simulink model "SensorModels"  (R2018b)
settings: Solver=VariableStepAuto  StartTime=0.0  StopTime=10.0  RelTol=1e-3
libraries: simulink x5
settings Model: Creator=Andrew  LastModifiedBy=Andrew

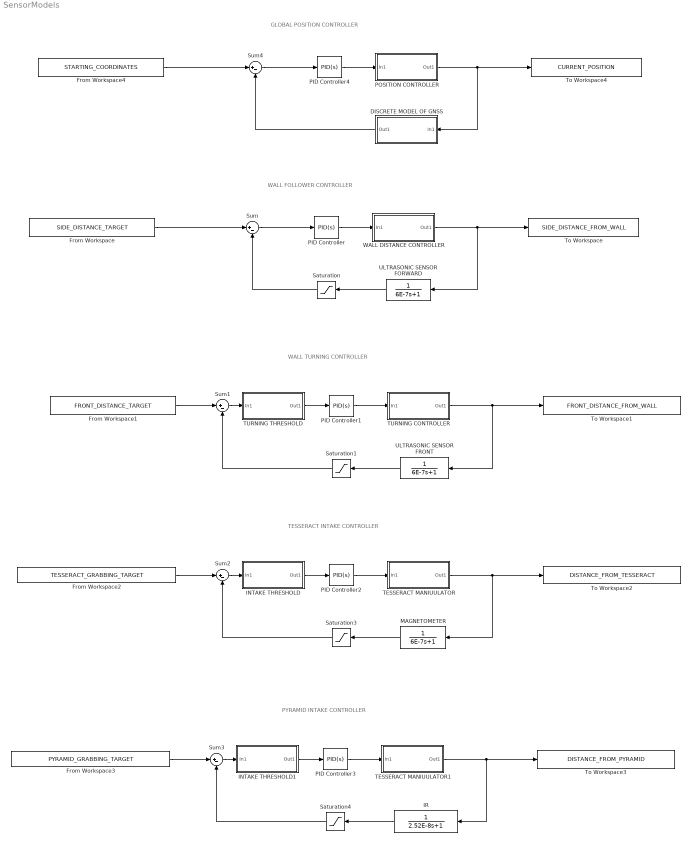
== system SensorModels ==
  note: WALL FOLLOWER CONTROLLER
  note: WALL TURNING CONTROLLER
  note: TESSERACT INTAKE CONTROLLER
  note: PYRAMID INTAKE CONTROLLER
  note: GLOBAL POSITION CONTROLLER
  DISCRETE MODEL OF GNSS : Subsystem
  From Workspace : FromWorkspace  VariableName=SIDE_DISTANCE_TARGET  SampleTime=0
  From Workspace1 : FromWorkspace  VariableName=FRONT_DISTANCE_TARGET  SampleTime=0
  From Workspace2 : FromWorkspace  VariableName=TESSERACT_GRABBING_TARGET  SampleTime=0
  From Workspace3 : FromWorkspace  VariableName=PYRAMID_GRABBING_TARGET  SampleTime=0
  From Workspace4 : FromWorkspace  VariableName=STARTING_COORDINATES  SampleTime=0
  INTAKE THRESHOLD : Subsystem
  INTAKE THRESHOLD1 : Subsystem
  IR : TransferFcn  Denominator=[2.52E-8 1]
  MAGNETOMETER : TransferFcn  Denominator=[6E-7 1]
  PID Controller{,1..4} (5 alike) : simulink/Continuous/PID Controller  Controller=PID  Form=Parallel  TimeDomain=Continuous-time  SampleTime=-1  IntegratorMethod=Forward Euler  FilterMethod=Forward Euler  ControllerParametersSource=internal  P=1  I=1  D=0  UseFilter=on  N=100  TunerSelectOption=Transfer Function Based (PID Tuner App)  InitialConditionSource=internal  InitialConditionForIntegrator=0  InitialConditionForFilter=0  DifferentiatorICPrevScaledInput=0  ExternalReset=none  TrackingMode=off  Kt=1  LimitOutput=off  UpperSaturationLimit=inf  LowerSaturationLimit=-inf  LinearizeAsGain=on  AntiWindupMode=none  Kb=1  POutMin=[]  POutMax=[]  IOutMin=[]  IOutMax=[]  DOutMin=[]  DOutMax=[]  NOutMin=[]  NOutMax=[]  SumOutMin=[]  SumOutMax=[]  SaturationOutMin=[]  SaturationOutMax=[]  PParamMin=[]  PParamMax=[]  IParamMin=[]  IParamMax=[]  DParamMin=[]  DParamMax=[]  NParamMin=[]  NParamMax=[]  KbParamMin=[]  KbParamMax=[]  KtParamMin=[]  KtParamMax=[]  KbOutMin=[]  KbOutMax=[]  KtOutMin=[]  KtOutMax=[]  IntegratorOutMin=[]  IntegratorOutMax=[]  FilterOutMin=[]  FilterOutMax=[]  SumI1OutMin=[]  SumI1OutMax=[]  SumI2OutMin=[]  SumI2OutMax=[]  SumI3OutMin=[]  SumI3OutMax=[]  SumI4OutMin=[]  SumI4OutMax=[]  SumDOutMin=[]  SumDOutMax=[]  DifferentiatorOutMin=[]  DifferentiatorOutMax=[]  FilterDiffOutCoefMin=[]  FilterDiffOutCoefMax=[]  ReciprocalOutMin=[]  ReciprocalOutMax=[]  SumDenOutMin=[]  SumDenOutMax=[]  SumNumOutMin=[]  SumNumOutMax=[]  DivideOutMin=[]  DivideOutMax=[]  IntegratorContinuousStateAttributes=''  IntegratorStateMustResolveToSignalObject=off  IntegratorRTWStateStorageClass=Auto  FilterContinuousStateAttributes=''  FilterStateMustResolveToSignalObject=off  FilterRTWStateStorageClass=Auto  ParallelPVariant=InternalParameters  IdealPVariant=Disabled  IVariant=InternalParameters  DVariant=InternalParameters  IntegratorVariant=Continuous  SatVariant=Disabled  AWVariant=Passthrough  PCopyVariant=Disabled  TRVariant=Disabled  FdbkBlocksVariant=Forward  IdealPFdbkVariant=Disabled  SatFdbkVariant=Disabled  DerivativeFilterVariant=ContFilter  NVariant=InternalParameters  NCopyVariant=Disabled  FilterICVariant=InternalICsFilter  IntegratorICVariant=InternalICs  ExternalResetVariant=Disabled  TRSumVariant=Passthrough  SumFdbkVariant=Disabled  SumVariant=Sum_PID
  POSITION CONTROLLER : Subsystem
  Saturation{,1,3..4} (4 alike) : Saturate
  Sum{,1..4} (5 alike) : Sum  Inputs=|+-
  TESSERACT MANIUULATOR : Subsystem
  TESSERACT MANIUULATOR1 : Subsystem
  TURNING CONTROLLER : Subsystem
  TURNING THRESHOLD : Subsystem
  To Workspace : ToWorkspace  VariableName=SIDE_DISTANCE_FROM_WALL  SaveFormat=Timeseries  SampleTime=-1
  To Workspace1 : ToWorkspace  VariableName=FRONT_DISTANCE_FROM_WALL  SaveFormat=Timeseries  SampleTime=-1
  To Workspace2 : ToWorkspace  VariableName=DISTANCE_FROM_TESSERACT  SaveFormat=Timeseries  SampleTime=-1
  To Workspace3 : ToWorkspace  VariableName=DISTANCE_FROM_PYRAMID  SaveFormat=Timeseries  SampleTime=-1
  To Workspace4 : ToWorkspace  VariableName=CURRENT_POSITION  SaveFormat=Timeseries  SampleTime=-1
  ULTRASONIC SENSOR FORWARD : TransferFcn  Denominator=[6E-7 1]
  ULTRASONIC SENSOR FRONT : TransferFcn  Denominator=[6E-7 1]
  WALL DISTANCE CONTROLLER : Subsystem
  wires:
  ULTRASONIC SENSOR FORWARD/1 -> Saturation/1
  Sum/1 -> PID Controller/1
  PID Controller/1 -> WALL DISTANCE CONTROLLER/1(In1)
  WALL DISTANCE CONTROLLER/1(Out1) -> To Workspace/1, ULTRASONIC SENSOR FORWARD/1
  From Workspace/1 -> Sum/1
  Sum1/1 -> TURNING THRESHOLD/1(In1)
  TURNING CONTROLLER/1(Out1) -> To Workspace1/1, ULTRASONIC SENSOR FRONT/1
  Saturation1/1 -> Sum1/2
  From Workspace1/1 -> Sum1/1
  ULTRASONIC SENSOR FRONT/1 -> Saturation1/1
  TURNING THRESHOLD/1(Out1) -> PID Controller1/1
  PID Controller1/1 -> TURNING CONTROLLER/1(In1)
  TESSERACT MANIUULATOR/1(Out1) -> To Workspace2/1, MAGNETOMETER/1
  MAGNETOMETER/1 -> Saturation3/1
  Saturation3/1 -> Sum2/2
  Sum2/1 -> INTAKE THRESHOLD/1(In1)
  PID Controller2/1 -> TESSERACT MANIUULATOR/1(In1)
  INTAKE THRESHOLD/1(Out1) -> PID Controller2/1
  From Workspace2/1 -> Sum2/1
  TESSERACT MANIUULATOR1/1(Out1) -> To Workspace3/1, IR/1
  From Workspace3/1 -> Sum3/1
  INTAKE THRESHOLD1/1(Out1) -> PID Controller3/1
  PID Controller3/1 -> TESSERACT MANIUULATOR1/1(In1)
  IR/1 -> Saturation4/1
  Saturation4/1 -> Sum3/2
  Sum3/1 -> INTAKE THRESHOLD1/1(In1)
  Saturation/1 -> Sum/2
  POSITION CONTROLLER/1(Out1) -> DISCRETE MODEL OF GNSS/1(In1), To Workspace4/1
  PID Controller4/1 -> POSITION CONTROLLER/1(In1)
  Sum4/1 -> PID Controller4/1
  From Workspace4/1 -> Sum4/1
  DISCRETE MODEL OF GNSS/1(Out1) -> Sum4/2

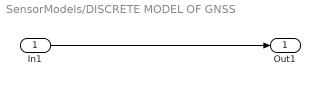
== system SensorModels/DISCRETE MODEL OF GNSS ==
  In1 : Inport
  Out1 : Outport
  wires:
  In1/1 -> Out1/1

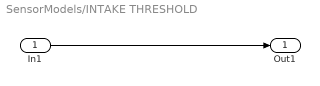
== system SensorModels/INTAKE THRESHOLD ==
  In1 : Inport
  Out1 : Outport
  wires:
  In1/1 -> Out1/1

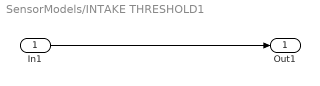
== system SensorModels/INTAKE THRESHOLD1 ==
  In1 : Inport
  Out1 : Outport
  wires:
  In1/1 -> Out1/1

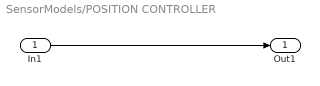
== system SensorModels/POSITION CONTROLLER ==
  In1 : Inport
  Out1 : Outport
  wires:
  In1/1 -> Out1/1

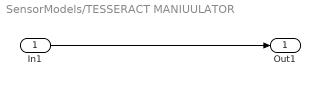
== system SensorModels/TESSERACT MANIUULATOR ==
  In1 : Inport
  Out1 : Outport
  wires:
  In1/1 -> Out1/1

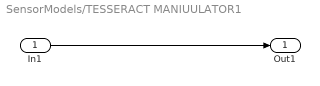
== system SensorModels/TESSERACT MANIUULATOR1 ==
  In1 : Inport
  Out1 : Outport
  wires:
  In1/1 -> Out1/1

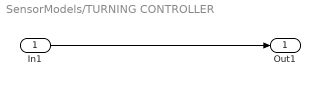
== system SensorModels/TURNING CONTROLLER ==
  In1 : Inport
  Out1 : Outport
  wires:
  In1/1 -> Out1/1

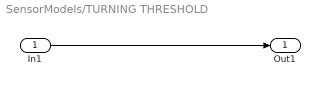
== system SensorModels/TURNING THRESHOLD ==
  In1 : Inport
  Out1 : Outport
  wires:
  In1/1 -> Out1/1

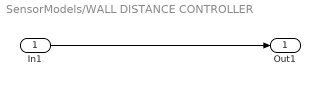
== system SensorModels/WALL DISTANCE CONTROLLER ==
  In1 : Inport
  Out1 : Outport
  wires:
  In1/1 -> Out1/1
